simulink model "untitled"  (R2023b)
settings: Solver=FixedStepAuto  StartTime=0.0  StopTime=10.0  FixedStep=1e-4  RelTol=1e-3
settings Model: DataDictionary=Clark_test.sldd  Creator=00033411  LastModifiedBy=00033411
settings OptimizationCC: DefaultParameterBehavior=Inlined  UseDivisionForNetSlopeComputation=on  GainParamInheritBuiltInType=on  UseFloatMulNetSlope=on  InlineInvariantSignals=on  PassReuseOutputArgsAs=Individual arguments  ZeroExternalMemoryAtStartup=off  ZeroInternalMemoryAtStartup=off  NoFixptDivByZeroProtection=on  EfficientFloat2IntCast=on  LifeSpan=1  OptimizeBlockOrder=speed  DifferentSizesBufferReuse=on  EfficientTunableParamExpr=on
settings DebuggingCC: ParameterPrecisionLossMsg=none  ParameterTunabilityLossMsg=error
settings HardwareCC: ProdBitPerPointer=32  ProdBitPerSizeT=32  ProdBitPerPtrDiffT=32  ProdLargestAtomicInteger=Long  ProdLargestAtomicFloat=Double  ProdWordSize=32  ProdLongLongMode=on  ProdHWDeviceType=ARM Compatible->ARM Cortex-M
settings SFSimCC: MATLABDynamicMemAlloc=off
settings RTWCC: Description=Embedded Coder  SystemTargetFile=ert.tlc  TemplateMakefile=ert_default_tmf  GenerateReport=on  LaunchReport=on
settings CodeAppCC: ForceParamTrailComments=on  IgnoreCustomStorageClasses=off  OperatorAnnotations=on  SimulinkDataObjDesc=on  SFDataObjDesc=on  CustomSymbolStrGlobalVar=rt$N$M  CustomSymbolStrType=$N$M  CustomSymbolStrFcn=$N$M$F  CustomSymbolStrMacro=$N$M  InsertBlockDesc=on
settings ERTTargetCC: TargetLangStandard=C99 (ISO)  CodeReplacementLibrary=ARM Cortex-M  GenerateSampleERTMain=on  IncludeMdlTerminateFcn=off  CombineSignalStateStructs=on  SupportAbsoluteTime=off  SupportNonFinite=off  SupportComplex=off  SupportNonInlinedSFcns=on  InlinedParameterPlacement=NonHierarchical  ERTCustomFileTemplate=example_file_process.tlc  ERTFilePackagingFormat=CompactWithDataFile

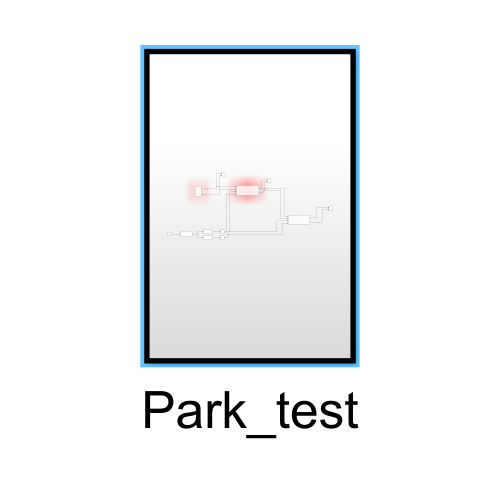
[thumbnail: Simulink's stored preview of the top-level diagram]
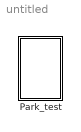
== system untitled ==
  Park_test : Subsystem  TreatAsAtomicUnit=on

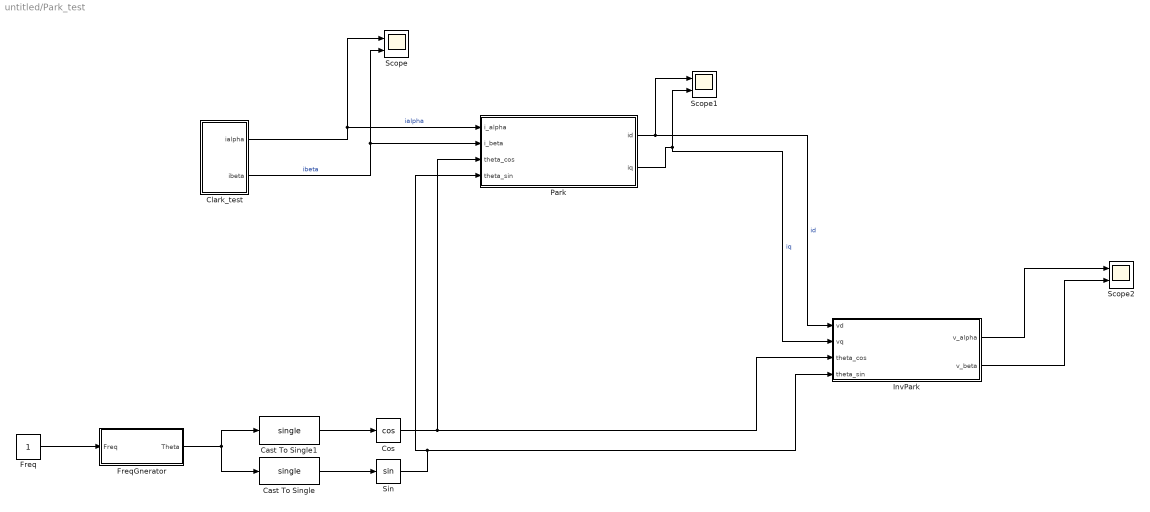
== system untitled/Park_test ==
  Cast To Single : DataTypeConversion  OutDataTypeStr=single  SaturateOnIntegerOverflow=off  RndMeth=Floor
  Cast To Single1 : DataTypeConversion  OutDataTypeStr=single  SaturateOnIntegerOverflow=off  RndMeth=Floor
  Clark_test : Subsystem  TreatAsAtomicUnit=on
  Cos : Trigonometry  Operator=cos
  Freq : Constant
  FreqGnerator : Subsystem
  InvPark : MATLAB Function  TreatAsAtomicUnit=on
  Park : MATLAB Function  TreatAsAtomicUnit=on
  Scope : Scope  NumInputPorts=2
  Scope1 : Scope  NumInputPorts=2
  Scope2 : Scope  NumInputPorts=2
  Sin : Trigonometry
  wires:
  InvPark/2(v_beta) -> Scope2/2
  Cos/1 -> InvPark/3(theta_cos), Park/3(theta_cos)
  Park/2(iq) -> Scope1/2, InvPark/2(vq)  "iq"
  Clark_test/1(ialpha) -> Scope/1, Park/1(i_alpha)  "ialpha"
  Freq/1 -> FreqGnerator/1(Freq)
  FreqGnerator/1(Theta) -> Cast To Single/1, Cast To Single1/1
  Cast To Single1/1 -> Cos/1
  Clark_test/2(ibeta) -> Scope/2, Park/2(i_beta)  "ibeta"
  Park/1(id) -> Scope1/1, InvPark/1(vd)  "id"
  Sin/1 -> InvPark/4(theta_sin), Park/4(theta_sin)
  Cast To Single/1 -> Sin/1
  InvPark/1(v_alpha) -> Scope2/1

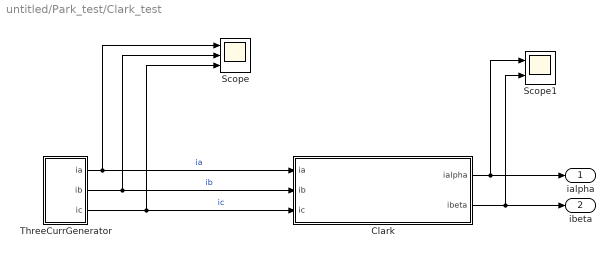
== system untitled/Park_test/Clark_test ==
  Clark : MATLAB Function  TreatAsAtomicUnit=on
  Scope : Scope  NumInputPorts=3
  Scope1 : Scope  NumInputPorts=2
  ThreeCurrGenerator : Subsystem
  ialpha : Outport
  ibeta : Outport  Port=2
  wires:
  ThreeCurrGenerator/2(ib) -> Clark/2(ib), Scope/2  "ib"
  ThreeCurrGenerator/3(ic) -> Clark/3(ic), Scope/3  "ic"
  Clark/1(ialpha) -> ialpha/1, Scope1/1
  Clark/2(ibeta) -> ibeta/1, Scope1/2
  ThreeCurrGenerator/1(ia) -> Clark/1(ia), Scope/1  "ia"

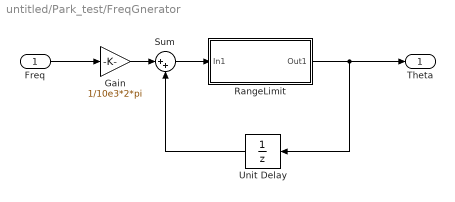
== system untitled/Park_test/FreqGnerator ==
  Freq : Inport
  Gain : Gain  Gain=1/10e3*2*pi
  RangeLimit : Subsystem
  Sum : Sum  Inputs=|++
  Unit Delay : UnitDelay  SampleTime=-1  HasFrameUpgradeWarning=on
  Theta : Outport
  wires:
  Freq/1 -> Gain/1
  RangeLimit/1(Out1) -> Unit Delay/1, Theta/1
  Gain/1 -> Sum/1
  Sum/1 -> RangeLimit/1(In1)
  Unit Delay/1 -> Sum/2

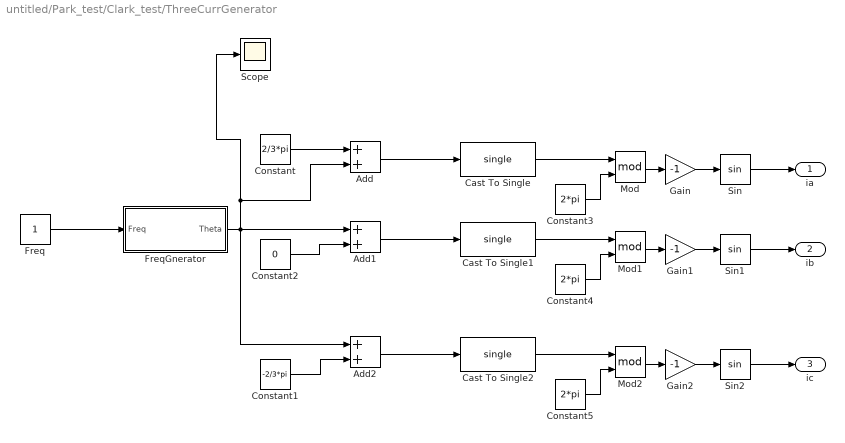
== system untitled/Park_test/Clark_test/ThreeCurrGenerator ==
  Add : Sum
  Add1 : Sum
  Add2 : Sum
  Cast To Single : DataTypeConversion  OutDataTypeStr=single  SaturateOnIntegerOverflow=off  RndMeth=Floor
  Cast To Single1 : DataTypeConversion  OutDataTypeStr=single  SaturateOnIntegerOverflow=off  RndMeth=Floor
  Cast To Single2 : DataTypeConversion  OutDataTypeStr=single  SaturateOnIntegerOverflow=off  RndMeth=Floor
  Constant : Constant  Value=2/3*pi
  Constant1 : Constant  Value=-2/3*pi
  Constant2 : Constant  Value=0
  Constant3 : Constant  Value=2*pi  OutDataTypeStr=single
  Constant4 : Constant  Value=2*pi  OutDataTypeStr=single
  Constant5 : Constant  Value=2*pi  OutDataTypeStr=single
  Freq : Constant
  FreqGnerator : Subsystem
  Gain : Gain  Gain=-1
  Gain1 : Gain  Gain=-1
  Gain2 : Gain  Gain=-1
  Mod : Math  Operator=mod
  Mod1 : Math  Operator=mod
  Mod2 : Math  Operator=mod
  Scope : Scope
  Sin : Trigonometry  ApproximationMethod=Lookup
  Sin1 : Trigonometry  ApproximationMethod=Lookup
  Sin2 : Trigonometry  ApproximationMethod=Lookup
  ia : Outport
  ib : Outport  Port=2
  ic : Outport  Port=3
  wires:
  Mod2/1 -> Gain2/1
  Sin/1 -> ia/1
  Add/1 -> Cast To Single/1
  Sin1/1 -> ib/1
  Freq/1 -> FreqGnerator/1(Freq)
  Cast To Single1/1 -> Mod1/1
  FreqGnerator/1(Theta) -> Scope/1, Add/2, Add2/1, Add1/1
  Cast To Single2/1 -> Mod2/1
  Gain2/1 -> Sin2/1
  Constant5/1 -> Mod2/2
  Add1/1 -> Cast To Single1/1
  Add2/1 -> Cast To Single2/1
  Sin2/1 -> ic/1
  Constant2/1 -> Add1/2
  Constant1/1 -> Add2/2
  Constant/1 -> Add/1
  Constant3/1 -> Mod/2
  Constant4/1 -> Mod1/2
  Cast To Single/1 -> Mod/1
  Gain1/1 -> Sin1/1
  Mod/1 -> Gain/1
  Gain/1 -> Sin/1
  Mod1/1 -> Gain1/1

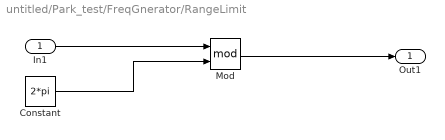
== system untitled/Park_test/FreqGnerator/RangeLimit ==
  In1 : Inport
  Constant : Constant  Value=2*pi
  Mod : Math  Operator=mod
  Out1 : Outport
  wires:
  In1/1 -> Mod/1
  Constant/1 -> Mod/2
  Mod/1 -> Out1/1

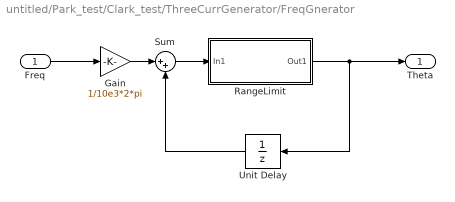
== system untitled/Park_test/Clark_test/ThreeCurrGenerator/FreqGnerator ==
  Freq : Inport
  Gain : Gain  Gain=1/10e3*2*pi
  RangeLimit : Subsystem
  Sum : Sum  Inputs=|++
  Unit Delay : UnitDelay  SampleTime=-1  HasFrameUpgradeWarning=on
  Theta : Outport
  wires:
  Freq/1 -> Gain/1
  RangeLimit/1(Out1) -> Unit Delay/1, Theta/1
  Gain/1 -> Sum/1
  Sum/1 -> RangeLimit/1(In1)
  Unit Delay/1 -> Sum/2

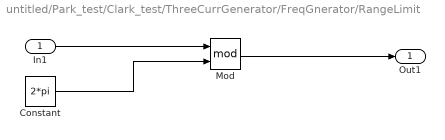
== system untitled/Park_test/Clark_test/ThreeCurrGenerator/FreqGnerator/RangeLimit ==
  In1 : Inport
  Constant : Constant  Value=2*pi
  Mod : Math  Operator=mod
  Out1 : Outport
  wires:
  In1/1 -> Mod/1
  Constant/1 -> Mod/2
  Mod/1 -> Out1/1

== matlab function untitled/Park_test/Park ==
  data: i_alpha input; id output; i_beta input; theta_cos input; theta_sin input; iq output
function [id, iq] = Park(i_alpha, i_beta, theta_cos, theta_sin)
% ==============================
% 标准Park变换 (αβ静止坐标系 → dq旋转坐标系)
% 输入：不使用theta！直接用预计算的 cosθ 和 sinθ
% i_alpha   : α轴电流
% i_beta    : β轴电流
% theta_cos : 电角度余弦值 cos(θ)
% theta_sin : 电角度正弦值 sin(θ)
% 输出：
% id : d轴励磁电流
% iq : q轴转矩电流
% ==============================

% 标准Park公式（直接代入cosθ/sinθ，无三角函数运算）
id = i_alpha * theta_cos + i_beta * theta_sin;
iq = -i_alpha * theta_sin + i_beta * theta_cos;
end

== matlab function untitled/Park_test/Clark_test/Clark ==
  data: ia input; ialpha output; ib input; ic input; ibeta output
function [ialpha, ibeta] = clark_current_equal_amp(ia, ib, ic)
% 电流等幅值Clark变换 (三相静止abc → 两相静止αβ)
% 输入：ia, ib, ic - 三相瞬时电流
% 输出：ialpha, ibeta - αβ轴电流分量

sqrt3 = sqrt(3); % 定义√3常数

% 等幅值变换核心公式
ialpha = (2*ia - ib - ic) / 3;  
ibeta  = sqrt3 * (ib - ic) / 3;  
end

== matlab function untitled/Park_test/InvPark ==
  data: vd input; v_alpha output; vq input; theta_cos input; theta_sin input; v_beta output
function [v_alpha, v_beta] = InvPark_Voltage(vd, vq, theta_cos, theta_sin)
% ==============================
% 电压型 反Park变换
% dq旋转坐标系 → αβ静止坐标系
% 输入：
%   vd        : d轴电压（电流环PI输出）
%   vq        : q轴电压（电流环PI输出）
%   theta_cos : 电角度余弦 cosθ
%   theta_sin : 电角度正弦 sinθ
% 输出：
%   v_alpha   : α轴静止电压
%   v_beta    : β轴静止电压
% ==============================

% 反Park标准公式（电压/电流通用）
v_alpha = vd * theta_cos - vq * theta_sin;
v_beta  = vd * theta_sin + vq * theta_cos;
end
